simulink model "Navigation"  (R2017a)
settings: Solver=FixedStepAuto  StartTime=0.0  StopTime=inf  FixedStep=0.01  RelTol=1e-3
settings Model: Creator=xiaodong  LastModifiedBy=xiaodong
settings DataIOCC: SaveFormat=Array  SaveOutput=off  SignalLogging=off  DSMLogging=off  SaveTime=off

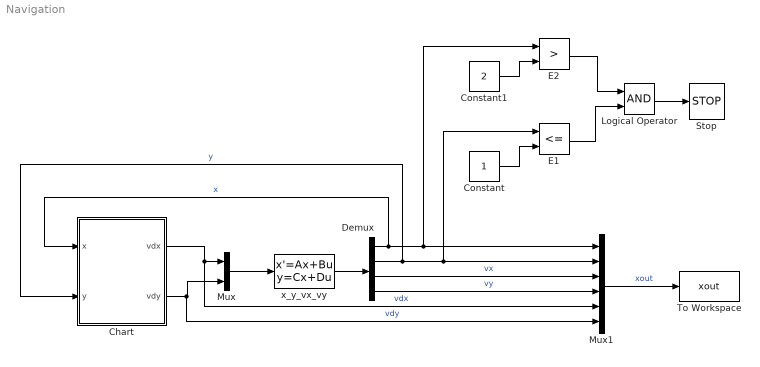
== system Navigation ==
  Chart : Stateflow chart  TreatAsAtomicUnit=on
  Constant : Constant
  Constant1 : Constant  Value=2
  Demux : Demux
  E1 : RelationalOperator  Operator=<=  OutDataTypeStr=boolean  RndMeth=Simplest
  E2 : RelationalOperator  Operator=>  OutDataTypeStr=boolean  RndMeth=Simplest
  Logical Operator : Logic  AllPortsSameDT=off  OutDataTypeStr=boolean
  Mux : Mux  Inputs=2
  Mux1 : Mux  Inputs=6
  Stop : Stop
  To Workspace : ToWorkspace  VariableName=xout  SampleTime=-1
  x_y_vx_vy : StateSpace  A=[0 0 1 0; 0 0 0 1; 0 0 -1.2 0.1; 0 0 0.1 -1.2]  B=-[0 0; 0 0; -1.2 0.1; 0.1 -1.2]  C=eye(4,4)  D=zeros(4,2)  X0="[1.60000000000000\t1.90000000000000\t-1.60000000000000\t0]"
  wires:
  Mux/1 -> x_y_vx_vy/1
  Chart/1(vdx) -> Mux1/5, Mux/1  "vdx"
  Chart/2(vdy) -> Mux1/6, Mux/2  "vdy"
  x_y_vx_vy/1 -> Demux/1
  Demux/1 -> Mux1/1, E2/1, Chart/1(x)  "x"
  Demux/2 -> Chart/2(y), Mux1/2, E1/1  "y"
  Demux/3 -> Mux1/3  "vx"
  Demux/4 -> Mux1/4  "vy"
  E1/1 -> Logical Operator/2
  E2/1 -> Logical Operator/1
  Logical Operator/1 -> Stop/1
  Constant/1 -> E1/2
  Constant1/1 -> E2/2
  Mux1/1 -> To Workspace/1  "xout"

== stateflow chart Navigation/Chart ==
  settings: stateMachineType=MOORE_MACHINE
  state sys
    state S1 [parallel]
      settings: executionOrder=2
      state S4
        label = 2;
        vdx = sin(label*pi/4);
        vdy = cos(label*pi/4);
      state S2
        label = 4;
        vdx = sin(label*pi/4);
        vdy = cos(label*pi/4);
      state S5
        label = 4;
        vdx = sin(label*pi/4);
        vdy = cos(label*pi/4);
      state S1
        label = 2;
        vdx = sin(label*pi/4);
        vdy = cos(label*pi/4);
      state S3
        label = 3;
        vdx = sin(label*pi/4);
        vdy = cos(label*pi/4);
      state A
      S2 -> S4 [order 2] : [c4==1]
      sys.S1.S1 -> S2 [order 1] : [c2==1]
      S4 -> S5 [order 2] : [c5==1]
      S4 -> S2 [order 1] : [c2==1]
      S2 -> sys.S1.S1 [order 1] : [c1==1]
      S5 -> S4 [order 2] : [c4==1]
      S4 -> S3 [order 3] : [c3==1]
      S3 -> S4 [order 4] : [c4==1]
      S3 -> S2 [order 3] : [c2==1]
      S2 -> S3 [order 3] : [c3==1]
      (default) -> sys.S1.S1
      sys.S1.S1 -> S3 [order 2] : [c3==1]
      S3 -> S5 [order 2] : [c5==1]
      S5 -> S3 [order 1] : [c3==1]
      S3 -> sys.S1.S1 [order 1] : [c1==1]
      sys.S1.S1 -> A [order 3] : [x>2]
      S5 -> A [order 3] : [y<=1]
    state Conditions [parallel]
      c1 = (x>=0 && x<=2 && y>=0 && y<=1);
      c2 = (x>=0 && x<=1 && y>1   && y<=2);
      c3 = (x>1   && x<=2 && y>1   && y<=2);
      c4 = (x>1   && x<=2 && y>2   && y<=3);
      c5 = (x>2   && x<=3 && y>1   && y<=3);
      settings: executionOrder=1
  (default) -> sys
  data: x input; y input; c1 local boolean =false; c2 local boolean =false; c3 local boolean =false; c4 local boolean =false; c5 local boolean =false; label local =2; vdx output; vdy output
